simulink model "Simple_pendulum_model"  (R2022b)
settings: Solver=VariableStepAuto  StartTime=0.0  StopTime=10.0  RelTol=1e-3
settings Model: Creator=NADA IBRAHIM  LastModifiedBy=NADA IBRAHIM

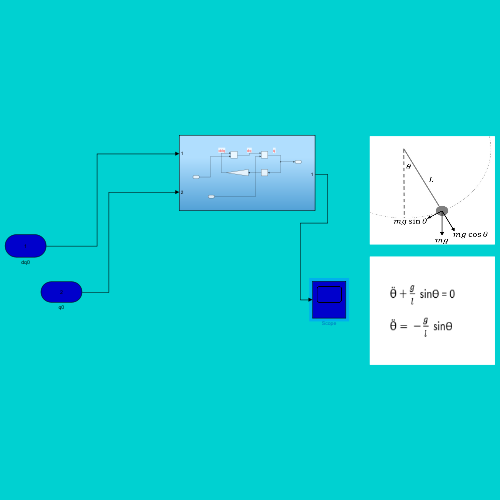
[thumbnail: Simulink's stored preview of the top-level diagram]
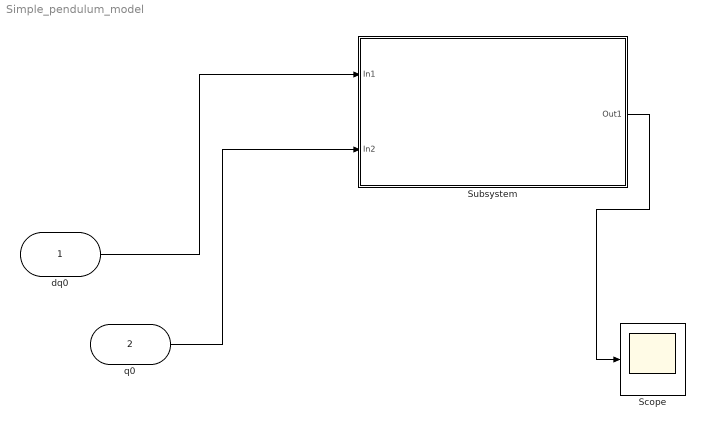
== system Simple_pendulum_model ==
  dq0 : Inport
  q0 : Inport  Port=2
  Scope : Scope
  Subsystem : Subsystem
  wires:
  dq0/1 -> Subsystem/1(In1)
  q0/1 -> Subsystem/2(In2)
  Subsystem/1(Out1) -> Scope/1

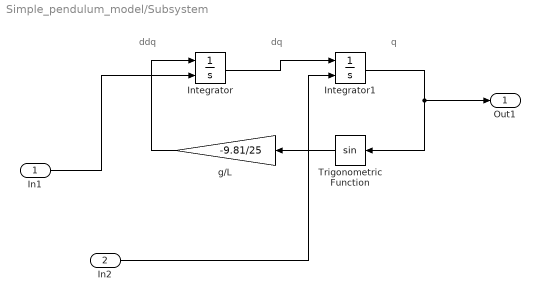
== system Simple_pendulum_model/Subsystem ==
  note: q
  note: dq
  note: ddq
  In1 : Inport
  In2 : Inport  Port=2
  Integrator : Integrator  InitialConditionSource=external
  Integrator1 : Integrator  InitialConditionSource=external
  Trigonometric Function : Trigonometry
  g/L : Gain  Gain=-9.81/25
  Out1 : Outport
  wires:
  Integrator/1 -> Integrator1/1
  In1/1 -> Integrator/2
  Integrator1/1 -> Out1/1, Trigonometric Function/1
  In2/1 -> Integrator1/2
  Trigonometric Function/1 -> g/L/1
  g/L/1 -> Integrator/1
